simulink model "Prob2"  (R2020b)
settings: Solver=VariableStepAuto  StartTime=0.0  StopTime=10.0  RelTol=1e-3
model workspace (MAT data in the model file):
  b = Simulink.Parameter
  b.Value = 350
  b.DataType = 'auto'
  b.Dimensions = [1 1]
  k1 = Simulink.Parameter
  k1.Value = 80000
  k1.DataType = 'auto'
  k1.Dimensions = [1 1]
  k2 = Simulink.Parameter
  k2.Value = 500000
  k2.DataType = 'auto'
  k2.Dimensions = [1 1]
  m1 = Simulink.Parameter
  m1.Value = 2500
  m1.DataType = 'auto'
  m1.Dimensions = [1 1]
  m2 = Simulink.Parameter
  m2.Value = 320
  m2.DataType = 'auto'
  m2.Dimensions = [1 1]
settings Model: Creator=shoun  LastModifiedBy=shoun

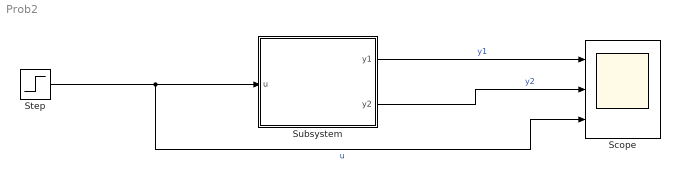
== system Prob2 ==
  Scope : Scope  NumInputPorts=3
  Step : Step  SampleTime=0
  Subsystem : Subsystem
  wires:
  Subsystem/1(y1) -> Scope/1  "y1"
  Subsystem/2(y2) -> Scope/2  "y2"
  Step/1 -> Scope/3, Subsystem/1(u)  "u"

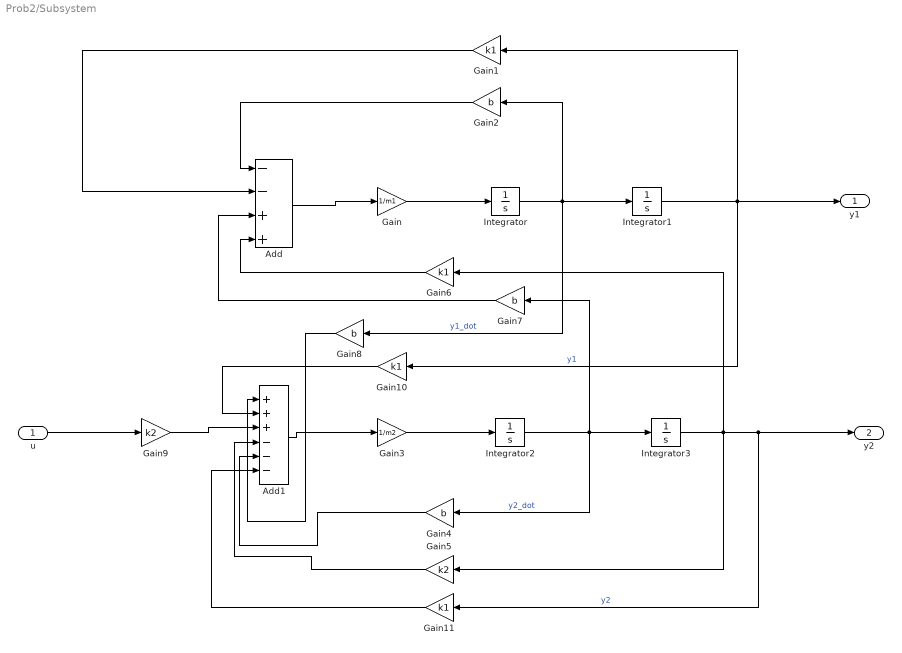
== system Prob2/Subsystem ==
  u : Inport
  Add : Sum  Inputs=--++
  Add1 : Sum  Inputs=+++---
  Gain : Gain  Gain=1/m1
  Gain{1,6,10..11} (4 alike) : Gain  Gain=k1
  Gain{2,4,7..8} (4 alike) : Gain  Gain=b
  Gain3 : Gain  Gain=1/m2
  Gain5 : Gain  Gain=k2
  Gain9 : Gain  Gain=k2
  Integrator{,1..3} (4 alike) : Integrator
  y1 : Outport
  y2 : Outport  Port=2
  wires:
  Integrator2/1 -> Gain7/1, Gain4/1, Integrator3/1  "y2_dot"
  Gain4/1 -> Add1/5
  Gain/1 -> Integrator/1
  Gain8/1 -> Add1/1
  Integrator1/1 -> y1/1, Gain10/1, Gain1/1  "y1"
  Add/1 -> Gain/1
  Gain1/1 -> Add/2
  u/1 -> Gain9/1
  Gain11/1 -> Add1/6
  Integrator/1 -> Gain8/1, Gain2/1, Integrator1/1  "y1_dot"
  Gain7/1 -> Add/3
  Gain2/1 -> Add/1
  Gain10/1 -> Add1/2
  Add1/1 -> Gain3/1
  Gain6/1 -> Add/4
  Gain9/1 -> Add1/3
  Integrator3/1 -> Gain6/1, Gain5/1, y2/1, Gain11/1  "y2"
  Gain5/1 -> Add1/4
  Gain3/1 -> Integrator2/1
